simulink model "sim_3"  (R2013b)
settings: Solver=ode45  StartTime=0.0  StopTime=10.0  RelTol=1e-3
settings Model: Creator=Ali  LastModifiedBy=Ali

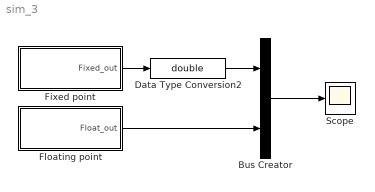
== system sim_3 ==
  Bus Creator : BusCreator  Inputs=2
  Data Type Conversion2 : DataTypeConversion  OutDataTypeStr=double
  Fixed point : Subsystem
  Floating point : Subsystem
  Scope : Scope
      settings: YMin=-1  YMax=1
  wires:
  Bus Creator/1 -> Scope/1
  Data Type Conversion2/1 -> Bus Creator/1
  Floating point/1(Float_out) -> Bus Creator/2
  Fixed point/1(Fixed_out) -> Data Type Conversion2/1

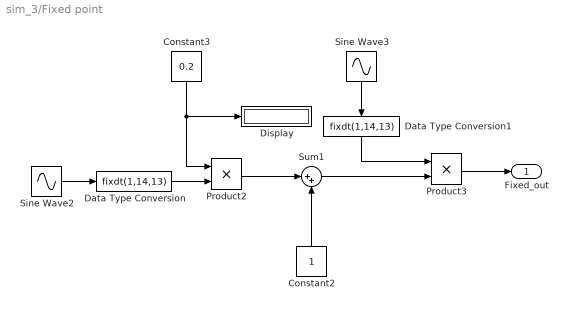
== system sim_3/Fixed point ==
  Constant2 : Constant  OutDataTypeStr=fixdt(1,9,8)
  Constant3 : Constant  Value=0.2  OutDataTypeStr=fixdt(1,9,8)
  Data Type Conversion : DataTypeConversion  OutDataTypeStr=fixdt(1,14,13)
  Data Type Conversion1 : DataTypeConversion  OutDataTypeStr=fixdt(1,14,13)
  Display : Display
  Product2 : Product  OutDataTypeStr=fixdt(1,10,8)
  Product3 : Product  OutDataTypeStr=fixdt(1,16,13)
  Sine Wave2 : Sin  Frequency=2*pi*94  Phase=pi/2  SampleTime=1/100e6
  Sine Wave3 : Sin  Frequency=2*pi*430e3  SampleTime=1/100e6
  Sum1 : Sum  Inputs=|++  OutDataTypeStr=fixdt(1,15,13)
  Fixed_out : Outport
  wires:
  Data Type Conversion/1 -> Product2/2
  Constant3/1 -> Product2/1, Display/1
  Product2/1 -> Sum1/1
  Sum1/1 -> Product3/2
  Sine Wave3/1 -> Data Type Conversion1/1
  Sine Wave2/1 -> Data Type Conversion/1
  Constant2/1 -> Sum1/2
  Data Type Conversion1/1 -> Product3/1
  Product3/1 -> Fixed_out/1

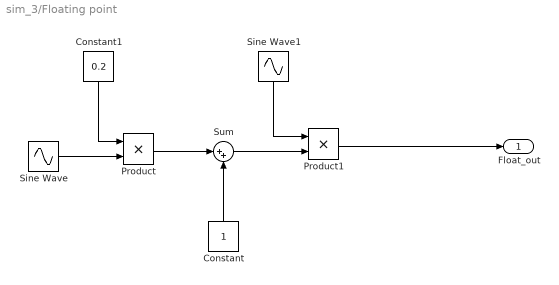
== system sim_3/Floating point ==
  Constant : Constant
  Constant1 : Constant  Value=0.2
  Product : Product
  Product1 : Product
  Sine Wave : Sin  Frequency=2*pi*94  Phase=pi/2  SampleTime=1/100e6
  Sine Wave1 : Sin  Frequency=2*pi*430e3  SampleTime=1/100e6
  Sum : Sum  Inputs=|++
  Float_out : Outport
  wires:
  Product1/1 -> Float_out/1
  Sine Wave/1 -> Product/2
  Constant1/1 -> Product/1
  Sine Wave1/1 -> Product1/1
  Product/1 -> Sum/1
  Sum/1 -> Product1/2
  Constant/1 -> Sum/2
